simulink model "Quadrature_Phase_Distance_Detection"  (R2016b)
settings: Solver=FixedStepDiscrete  StartTime=0.0  StopTime=inf  RelTol=1e-3
libraries: simulink x1
settings Model: Creator=zahid  LastModifiedBy=z_amin
settings SolverCC: AutoInsertRateTranBlk=on
settings DataIOCC: LimitDataPoints=on  SaveOutput=off  SignalLogging=off  SaveTime=off
settings OptimizationCC: LifeSpan=inf
settings DebuggingCC: AlgebraicLoopMsg=error  SingleTaskRateTransMsg=error  AllowSymbolicDim=off  SFUnexpectedBacktrackingDiag=warning  SFNoUnconditionalDefaultTransitionDiag=warning  SFExecutionAtInitializationDiag=none
settings GRTTargetCC: TargetLangStandard=C89/C90 (ANSI)  GeneratePreprocessorConditionals=Disable all
settings ConfigComp: CovMetricSettings=dw  CovHtmlReporting=on  CovSaveCumulativeToWorkspaceVar=on  CovSaveSingleToWorkspaceVar=on  CovExternalEMLEnable=off

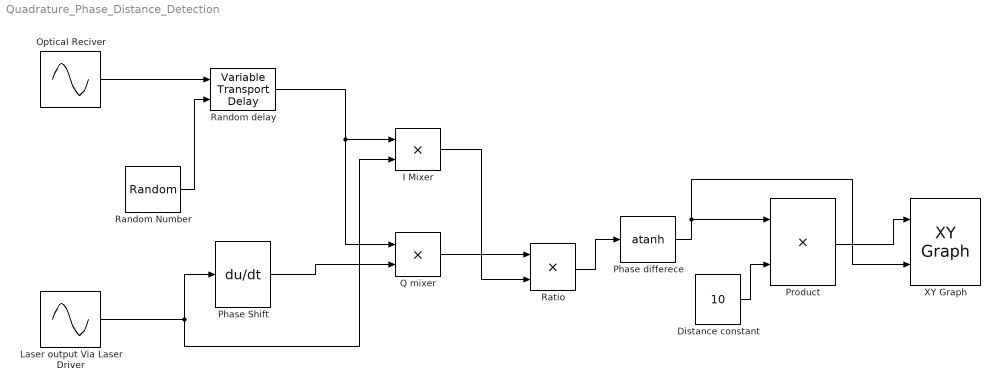
== system Quadrature_Phase_Distance_Detection ==
  Distance constant : Constant  Value=10
  I Mixer : Product
  Laser output Via Laser Driver : Sin  Frequency=10  SampleTime=0
  Optical Reciver : Sin  Frequency=10  SampleTime=0
  Phase Shift : Derivative
  Phase differece : Trigonometry  Operator=atanh  OutputSignalType=real
  Product : Product
  Q mixer : Product
  Random Number : RandomNumber  Mean=1  SampleTime=0.1
  "Random delay " : VariableTransportDelay  MaximumDelay=10
  Ratio : Product
  XY Graph : simulink/Sinks/XY Graph  xmin=-1  xmax=25  ymin=-1  ymax=3  st=-1
  wires:
  Distance constant/1 -> Product/2
  Optical Reciver/1 -> "Random delay "/1
  Random Number/1 -> "Random delay "/2
  Laser output Via Laser Driver/1 -> I Mixer/2, Phase Shift/1
  "Random delay "/1 -> Q mixer/1, I Mixer/1
  Phase Shift/1 -> Q mixer/2
  Q mixer/1 -> Ratio/1
  I Mixer/1 -> Ratio/2
  Ratio/1 -> Phase differece/1
  Phase differece/1 -> Product/1, XY Graph/2
  Product/1 -> XY Graph/1
